simulink model "sim_suspension_external_function"  (R2024a)
settings: Solver=ode45  StartTime=0.0  StopTime=3  MaxStep=1e-3  RelTol=1e-3
undefined symbols (not defined in the file): k, m, r, road_excitation_amplitude, road_excitation_omega, v0, x0
settings Model: Creator=ArrigonDell  LastModifiedBy=Bocchio
settings SolverCC: AlgebraicLoopSolver=TrustRegion
settings DataIOCC: ReturnWorkspaceOutputs=off
settings DebuggingCC: UnconnectedInputMsg=warning  UnconnectedOutputMsg=warning  UnconnectedLineMsg=warning  ArithmeticOperatorsInVariantConditions=warning
settings ModelReferenceCC: EnableRefExpFcnMdlSchedulingChecks=on
settings SFSimCC: SimUseLocalCustomCode=off  CustomCodeUndefinedFunction=UseInterfaceOnly
settings RTWCC: RTWUseLocalCustomCode=off  GPUComputeCapability=3.5  DLArmComputeVersion=19.05

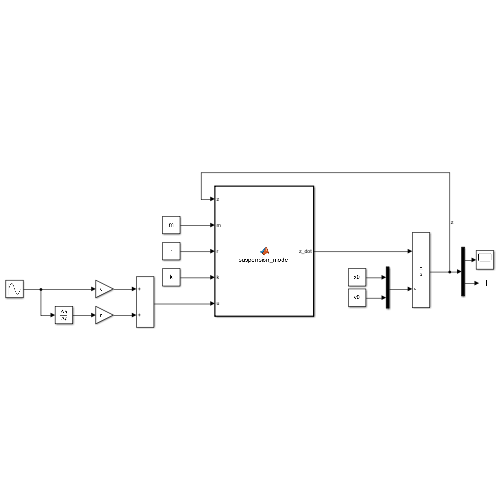
[thumbnail: Simulink's stored preview of the top-level diagram]
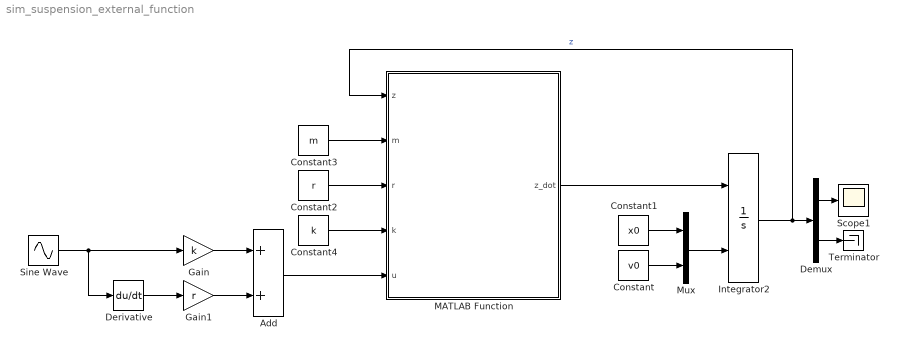
== system sim_suspension_external_function ==
  Add : Sum
  Constant : Constant  Value=v0
  Constant1 : Constant  Value=x0
  Constant2 : Constant  Value=r
  Constant3 : Constant  Value=m
  Constant4 : Constant  Value=k
  Demux : Demux  Outputs=2
  Derivative : Derivative
  Gain : Gain  Gain=k
  Gain1 : Gain  Gain=r
  Integrator2 : Integrator  InitialConditionSource=external
  MATLAB Function : MATLAB Function  TreatAsAtomicUnit=on
  Mux : Mux  Inputs=2
  Scope1 : Scope
  Sine Wave : Sin  Amplitude=road_excitation_amplitude  Frequency=road_excitation_omega  SampleTime=0
  Terminator : Terminator
  wires:
  Add/1 -> MATLAB Function/5(u)
  Derivative/1 -> Gain1/1
  Sine Wave/1 -> Gain/1, Derivative/1
  Gain/1 -> Add/1
  Gain1/1 -> Add/2
  Constant2/1 -> MATLAB Function/3(r)
  Constant3/1 -> MATLAB Function/2(m)
  Constant4/1 -> MATLAB Function/4(k)
  Constant1/1 -> Mux/1
  Constant/1 -> Mux/2
  MATLAB Function/1(z_dot) -> Integrator2/1
  Mux/1 -> Integrator2/2
  Integrator2/1 -> MATLAB Function/1(z), Demux/1  "z"
  Demux/1 -> Scope1/1
  Demux/2 -> Terminator/1

== matlab function sim_suspension_external_function/MATLAB Function ==
  data: z input; m input; r input; k input; z_dot output; u input
%===================================================================%
%                                                                   %
%   Vehicle suspension model for simulink                           %
%                                                                   %
%===================================================================%

function z_dot  = suspension_model(z, m, r, k, u)

z_dot = zeros(2, 1);

z_dot(1, 1) = z(2);
z_dot(2, 1) = -r/m * z(2) + ...
    -k/m * z(1) + ...
    +1/m * u;

end
